simulink model "sampleModel104"  (R2021b)
settings: Solver=VariableStepAuto  StartTime=0.0  StopTime=10.0  RelTol=1e-3
undefined symbols (not defined in the file or in its folder): Newton, Raphson
libraries: simulink x17, slpidlib x1
settings Model: Creator=user  LastModifiedBy=user

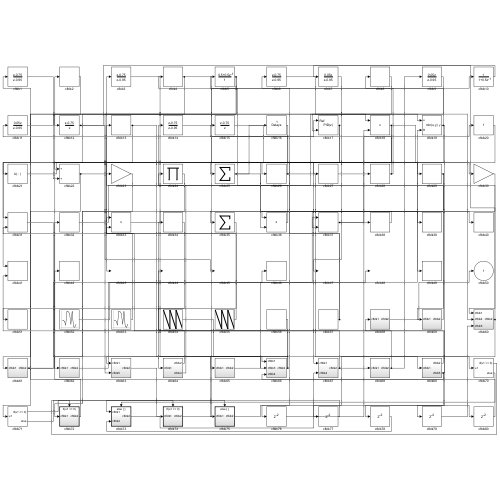
[thumbnail: Simulink's stored preview of the top-level diagram]
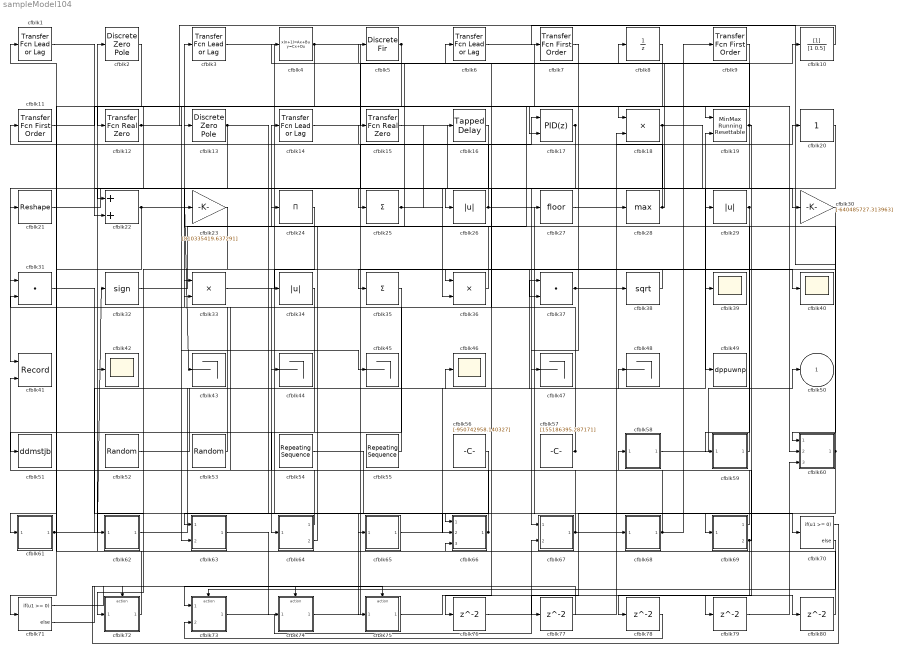
== system sampleModel104 ==
  cfblk{1,3,6,14} (4 alike) : simulink/Discrete/Transfer Fcn Lead or Lag  PoleZ=0.95  ZeroZ=0.75  ICPrevOutput=0.0  ICPrevInput=0.0  DoSatur=off
      settings: SourceProductBaseCode=SL
  cfblk10 : DiscreteFilter  SampleTime=1
  cfblk11 : simulink/Discrete/Transfer Fcn First Order  PoleZ=0.95  ICPrevOutput=0.0  DoSatur=off
  cfblk12 : simulink/Discrete/Transfer Fcn Real Zero  ZeroZ=0.75  ICPrevInput=0.0  DoSatur=off
      settings: SourceProductBaseCode=SL
  cfblk13 : DiscreteZeroPole  Poles=[0 0.5]  Gain=1
  cfblk15 : simulink/Discrete/Transfer Fcn Real Zero  ZeroZ=0.75  ICPrevInput=0.0  DoSatur=off
      settings: SourceProductBaseCode=SL
  cfblk16 : simulink/Discrete/Tapped Delay  vinit=0.0  samptime=-1  NumDelays=1  DelayOrder=Oldest  includeCurrent=off
  cfblk17 : slpidlib/PID Controller (2DOF)  Controller=PID  Form=Parallel  TimeDomain=Discrete-time  UseExternalTs=off  SampleTime=1  IntegratorMethod=Forward Euler  FilterMethod=Forward Euler  ControllerParametersSource=internal  P=1  I=1  D=0  UseFilter=on  N=100  b=1  c=1  TunerSelectOption=Transfer Function Based (PID Tuner App)  InitialConditionSource=internal  InitialConditionForIntegrator=0  InitialConditionForFilter=0  DifferentiatorICPrevScaledInput=0  ExternalReset=none  TrackingMode=off  Kt=1  LimitOutput=off  SatLimitsSource=internal  UpperSaturationLimit=inf  LowerSaturationLimit=-inf  LinearizeAsGain=off  AntiWindupMode=none  Kb=1  POutMin=[]  POutMax=[]  IOutMin=[]  IOutMax=[]  DOutMin=[]  DOutMax=[]  NOutMin=[]  NOutMax=[]  bOutMin=[]  bOutMax=[]  cOutMin=[]  cOutMax=[]  SumOutMin=[]  SumOutMax=[]  SaturationOutMin=[]  SaturationOutMax=[]  PParamMin=[]  PParamMax=[]  IParamMin=[]  IParamMax=[]  DParamMin=[]  DParamMax=[]  NParamMin=[]  NParamMax=[]  bParamMin=[]  bParamMax=[]  cParamMin=[]  cParamMax=[]  KbParamMin=[]  KbParamMax=[]  KtParamMin=[]  KtParamMax=[]  KbOutMin=[]  KbOutMax=[]  KtOutMin=[]  KtOutMax=[]  IntegratorOutMin=[]  IntegratorOutMax=[]  FilterOutMin=[]  FilterOutMax=[]  SumI1OutMin=[]  SumI1OutMax=[]  SumI2OutMin=[]  SumI2OutMax=[]  SumI3OutMin=[]  SumI3OutMax=[]  SumI4OutMin=[]  SumI4OutMax=[]  SumDOutMin=[]  SumDOutMax=[]  Sum1OutMin=[]  Sum1OutMax=[]  Sum2OutMin=[]  Sum2OutMax=[]  Sum3OutMin=[]  Sum3OutMax=[]  DifferentiatorOutMin=[]  DifferentiatorOutMax=[]  FilterDiffOutCoefMin=[]  FilterDiffOutCoefMax=[]  ReciprocalOutMin=[]  ReciprocalOutMax=[]  SumDenOutMin=[]  SumDenOutMax=[]  SumNumOutMin=[]  SumNumOutMax=[]  DivideOutMin=[]  DivideOutMax=[]  UdiffTsProdOutMin=[]  UdiffTsProdOutMax=[]  NTsProdOutMin=[]  NTsProdOutMax=[]  UintegralTsProdOutMin=[]  UintegralTsProdOutMax=[]  UngainTsProdOutMin=[]  UngainTsProdOutMax=[]  IntegratorContinuousStateAttributes=''  IntegratorStateMustResolveToSignalObject=off  IntegratorRTWStateStorageClass=Auto  FilterContinuousStateAttributes=''  FilterStateMustResolveToSignalObject=off  FilterRTWStateStorageClass=Auto  ParallelPVariant=InternalParameters  IdealPVariant=Disabled  IVariant=InternalParameters  DVariant=InternalParameters  bVariant=InternalParameters  cVariant=InternalParameters  IntegratorVariant=Discrete  SatVariant=Disabled  AWVariant=Passthrough  PCopyVariant=Disabled  TRVariant=Disabled  FdbkBlocksVariant=Forward  IdealPFdbkVariant=Disabled  SatFdbkVariant=Disabled  DerivativeFilterVariant=ForwardEulerFilter  NVariant=InternalParameters  NCopyVariant=Disabled  FilterICVariant=InternalICsFilter  IntegratorICVariant=InternalICs  ExternalResetVariant=Disabled  TRSumVariant=Passthrough  SumFdbkVariant=Disabled  SumVariant=Sum_PID  TsampFilterVariant=InternalTs  TsampNgainVariant=Passthrough  TsampIntegralVariant=Passthrough  ExternalSaturationOutDataTypeStr=Inherit: Same as second input
      settings: SourceProductBaseCode=SL
  cfblk18 : Product  Inputs=**
  cfblk19 : simulink/Math Operations/MinMax Running Resettable  Function=min  vinit=0.0
  cfblk2 : DiscreteZeroPole  Poles=[0 0.5]  Gain=1
  cfblk20 : simulink/Math Operations/Slider Gain  gain=1  low=0  high=2
  cfblk21 : Reshape
  cfblk22 : Sum
  cfblk23 : Gain  Gain=[810335419.637291]
  cfblk24 : Product  Inputs=*
  cfblk25 : Sum  Inputs=+
  cfblk26 : Abs
  cfblk27 : Rounding
  cfblk28 : MinMax  Function=max
  cfblk29 : Abs
  cfblk30 : Gain  Gain=[-640485727.313963]
  cfblk31 : DotProduct  InputSameDT=on  OutDataTypeStr=Inherit: Inherit via internal rule
  cfblk32 : Signum
  cfblk33 : Product
  cfblk34 : Abs
  cfblk35 : Sum  Inputs=+
  cfblk36 : Product  Inputs=**
  cfblk37 : DotProduct  InputSameDT=on  OutDataTypeStr=Inherit: Inherit via internal rule
  cfblk38 : Sqrt  SaturateOnIntegerOverflow=on
  cfblk{39..40,42,46} (4 alike) : Scope
  cfblk4 : DiscreteStateSpace
  cfblk41 : Record  FileSettingsInternal="{\"entries\":[{\"content\":{\"excelSettings\":{\"content\":{},\"type\":\"Streamout.ExcelSettings\"}},\"type\":\"Streamout.FileSettingStorage\",\"uuid\":\"84cf82fa-35bb-4254-a1fc-1f6b5955f86e\"}],\"packageUris\":[\"http://schema.mathworks.com/mf0/streamout_blocks/R2020a\"],\"version\":\"1.0\"}"  Layout=[1 1]  SignalsInternal="{\"entries\":[{\"content\":{\"signals\":[{\"content\":{\"blockPath\":[\"sampleModel104/cfblk41\"],\"channel\":[],\"dimensions\":[1],\"domain\":\"sampleModel104/cfblk41\",\"lineColor\":\"#a2142f\",\"plots\":[1],\"port\":1,\"sid\":[\"\"],\"signalID\":3732,\"signalName\":\"cfblk16\"},\"type\":\"RecordBlkView.Signal\",\"uuid\":\"75152f1e-4c02-4af2-84cf-784db9ba61d4\"},{\"content\":{\"blockPath\":[\"sampleModel104/cfblk41\"],\"channel\":[],\"dimensions\":[1],\"domain\":\"sampleModel104/cfblk41\",\"lineColor\":\"#139fff\",\"plots\":[1],\"port\":2,\"sid\":[\"\"],\"signalID\":3736,\"signalName\":\"cfblk66\"},\"type\":\"RecordBlkView.Signal\",\"uuid\":\"7964c5ee-3da1-484c-b3b6-d9e0f74eaa61\"}]},\"type\":\"RecordBlkView.InputSignals\",\"uuid\":\"6aa1200e-81fa-4e57-8f02-0c25f67a03be\"}],\"packageUris\":[\"http://schema.mathworks.com/mf0/streamout_blocks/R2020a\"],\"version\":\"1.0\"}"  VisualizationBindings="{\"xyplotplugin\":{\"info\":[{\"series\":[{\"bindingParametersList\":[{\"parameter\":\"X-Axis\",\"signalID\":3732,\"signalName\":\"cfblk16\"},{\"parameter\":\"Y-Axis\",\"signalID\":3736,\"signalName\":\"cfblk66\"}],\"seriesID\":3868}],\"subplotID\":1}]}}"  CompatibilityTag=XY
  cfblk{43..45,47..48} (5 alike) : Terminator
  cfblk49 : ToWorkspace  VariableName=dppuwnp  SaveFormat=Timeseries  SampleTime=-1
  cfblk5 : DiscreteFir  SampleTime=1
  cfblk51 : ToWorkspace  VariableName=ddmstjb  SaveFormat=Timeseries  SampleTime=-1
  cfblk52 : RandomNumber  Mean=[-16667.436370]  Variance=[47383.574054]  Seed=[56841479.000000]  SampleTime=0.1
  cfblk53 : RandomNumber  Mean=[25600.008098]  Variance=[37838.678242]  Seed=[330531999.000000]  SampleTime=0.1
  cfblk54 : simulink/Sources/Repeating Sequence  rep_seq_t=[0 2]  rep_seq_y=[249633370.551990, -336076107.817194]
  cfblk55 : simulink/Sources/Repeating Sequence  rep_seq_t=[0 2]  rep_seq_y=[799947842.512021, 579171463.259229]
  cfblk56 : Constant  Value=[-950742958.140327]  SampleTime=1
  cfblk57 : Constant  Value=[155186395.287171]  SampleTime=1
  cfblk58 : Subsystem
  cfblk59 : Subsystem
  cfblk60 : Subsystem
  cfblk61 : Subsystem
  cfblk62 : Subsystem
  cfblk63 : Subsystem
  cfblk64 : Subsystem
  cfblk65 : Subsystem
  cfblk66 : Subsystem
  cfblk67 : Subsystem
  cfblk68 : Subsystem
  cfblk69 : Subsystem
  cfblk7 : simulink/Discrete/Transfer Fcn First Order  PoleZ=0.95  ICPrevOutput=0.0  DoSatur=off
  cfblk70 : If  IfExpression=u1 >= 0  SampleTime=1
  cfblk71 : If  IfExpression=u1 >= 0  SampleTime=1
  cfblk72 : Subsystem  TreatAsAtomicUnit=on
  cfblk73 : Subsystem  TreatAsAtomicUnit=on
  cfblk74 : Subsystem  TreatAsAtomicUnit=on
  cfblk75 : Subsystem  TreatAsAtomicUnit=on
  cfblk{76..80} (5 alike) : Delay  SampleTime=1
  cfblk8 : UnitDelay  HasFrameUpgradeWarning=on
  cfblk9 : simulink/Discrete/Transfer Fcn First Order  PoleZ=0.95  ICPrevOutput=0.0  DoSatur=off
  cfblk50 : Outport
  wires:
  cfblk18/1 -> cfblk67/1(cfblk1), cfblk30/1, cfblk23/1
  cfblk16/1 -> cfblk41/1
  cfblk33/1 -> cfblk40/1
  cfblk32/1 -> cfblk19/1
  cfblk73/1(cfblk2) -> cfblk67/2(cfblk4)
  cfblk3/1 -> cfblk66/1(cfblk1)
  cfblk74/1(cfblk2) -> cfblk17/1
  cfblk17/1 -> cfblk31/1, cfblk76/1
  cfblk66/1(cfblk2) -> cfblk41/2, cfblk63/1(cfblk1)
  cfblk27/1 -> cfblk28/1
  cfblk72/1(cfblk2) -> cfblk2/1
  cfblk26/1 -> cfblk69/1(cfblk1), cfblk15/1
  cfblk36/1 -> cfblk3/1
  cfblk55/1 -> cfblk31/2
  cfblk7/1 -> cfblk47/1
  cfblk1/1 -> cfblk27/1
  cfblk59/1(cfblk2) -> cfblk14/1
  cfblk28/1 -> cfblk11/1, cfblk8/1
  cfblk19/1 -> cfblk26/1, cfblk4/1, cfblk79/1
  cfblk69/1(cfblk2) -> cfblk34/1
  cfblk69/2(cfblk5) -> cfblk58/1(cfblk1), cfblk66/3(cfblk4), cfblk78/1
  cfblk2/1 -> cfblk12/1
  cfblk12/1 -> cfblk60/1(cfblk1), cfblk45/1
  cfblk20/1 -> cfblk25/1
  cfblk61/1(cfblk2) -> cfblk32/1, cfblk46/1
  cfblk9/1 -> cfblk17/2
  cfblk54/1 -> cfblk66/2(cfblk3)
  cfblk52/1 -> cfblk19/2
  cfblk57/1 -> cfblk6/1, cfblk24/1
  cfblk56/1 -> cfblk75/1(cfblk1)
  cfblk60/1(cfblk2) -> cfblk5/1, cfblk77/1
  cfblk4/1 -> cfblk21/1, cfblk36/2
  cfblk68/1(cfblk2) -> cfblk44/1, cfblk9/1
  cfblk15/1 -> cfblk49/1
  cfblk65/1(cfblk2) -> cfblk48/1
  cfblk22/1 -> cfblk43/1, cfblk71/1
  cfblk38/1 -> cfblk35/1
  cfblk11/1 -> cfblk18/1
  cfblk53/1 -> cfblk13/1
  cfblk6/1 -> cfblk60/2(cfblk4)
  cfblk5/1 -> cfblk61/1(cfblk1), cfblk63/2(cfblk5)
  cfblk31/1 -> cfblk65/1(cfblk1)
  cfblk13/1 -> cfblk70/1, cfblk22/2
  cfblk25/1 -> cfblk39/1, cfblk16/1
  cfblk21/1 -> cfblk29/1
  cfblk62/1(cfblk2) -> cfblk37/1
  cfblk64/1(cfblk2) -> cfblk33/1
  cfblk30/1 -> cfblk36/1
  cfblk29/1 -> cfblk37/2, cfblk59/1(cfblk1)
  cfblk34/1 -> cfblk51/1
  cfblk37/1 -> cfblk38/1, cfblk20/1
  cfblk24/1 -> cfblk62/1(cfblk1)
  cfblk35/1 -> cfblk64/1(cfblk1)
  cfblk63/1(cfblk2) -> cfblk74/1(cfblk1)
  cfblk64/2(cfblk4) -> cfblk33/2
  cfblk8/1 -> cfblk22/1
  cfblk67/1(cfblk2) -> cfblk68/1(cfblk1), cfblk42/1
  cfblk23/1 -> cfblk72/1(cfblk1)
  cfblk14/1 -> cfblk10/1
  cfblk10/1 -> cfblk7/1
  cfblk58/1(cfblk2) -> cfblk50/1
  cfblk70/1 -> cfblk72/Action
  cfblk70/2 -> cfblk73/Action
  cfblk71/1 -> cfblk74/Action
  cfblk71/2 -> cfblk75/Action
  cfblk76/1 -> cfblk18/2
  cfblk77/1 -> cfblk73/1(cfblk1)
  cfblk78/1 -> cfblk73/2(cfblk4)
  cfblk79/1 -> cfblk60/3(cfblk5)
  cfblk75/1(cfblk2) -> cfblk80/1
  cfblk80/1 -> cfblk1/1

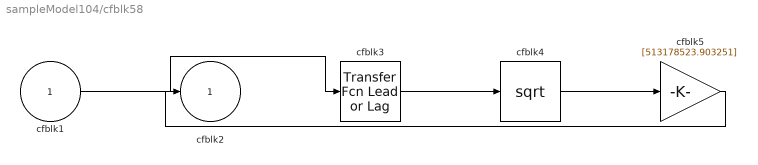
== system sampleModel104/cfblk58 ==
  cfblk1 : Inport
  cfblk3 : simulink/Discrete/Transfer Fcn Lead or Lag  PoleZ=0.95  ZeroZ=0.75  ICPrevOutput=0.0  ICPrevInput=0.0  DoSatur=off
      settings: SourceProductBaseCode=SL
  cfblk4 : Sqrt  SaturateOnIntegerOverflow=on
  cfblk5 : Gain  Gain=[513178523.903251]
  cfblk2 : Outport
  wires:
  cfblk3/1 -> cfblk4/1
  cfblk4/1 -> cfblk5/1
  cfblk1/1 -> cfblk3/1
  cfblk5/1 -> cfblk2/1

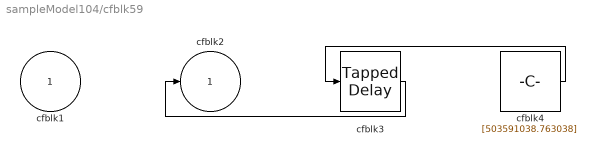
== system sampleModel104/cfblk59 ==
  cfblk1 : Inport
  cfblk3 : simulink/Discrete/Tapped Delay  vinit=0.0  samptime=-1  NumDelays=1  DelayOrder=Oldest  includeCurrent=off
  cfblk4 : Constant  Value=[503591038.763038]  SampleTime=1
  cfblk2 : Outport
  wires:
  cfblk4/1 -> cfblk3/1
  cfblk3/1 -> cfblk2/1

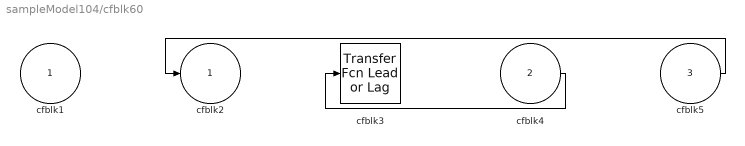
== system sampleModel104/cfblk60 ==
  cfblk1 : Inport
  cfblk4 : Inport  Port=2
  cfblk5 : Inport  Port=3
  cfblk3 : simulink/Discrete/Transfer Fcn Lead or Lag  PoleZ=0.95  ZeroZ=0.75  ICPrevOutput=0.0  ICPrevInput=0.0  DoSatur=off
      settings: SourceProductBaseCode=SL
  cfblk2 : Outport
  wires:
  cfblk5/1 -> cfblk2/1
  cfblk4/1 -> cfblk3/1

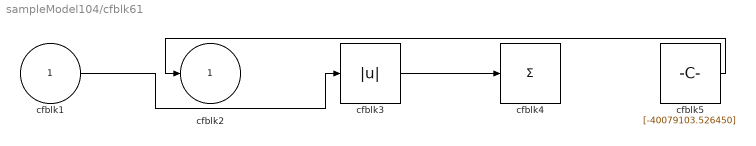
== system sampleModel104/cfblk61 ==
  cfblk1 : Inport
  cfblk3 : Abs
  cfblk4 : Sum  Inputs=+
  cfblk5 : Constant  Value=[-40079103.526450]  SampleTime=1
  cfblk2 : Outport
  wires:
  cfblk5/1 -> cfblk2/1
  cfblk1/1 -> cfblk3/1
  cfblk3/1 -> cfblk4/1

== system sampleModel104/cfblk62 ==
  cfblk1 : Inport
  cfblk3 : UnitDelay  HasFrameUpgradeWarning=on
  cfblk4 : Trigonometry
  cfblk2 : Outport
  wires:
  cfblk4/1 -> cfblk2/1
  cfblk1/1 -> cfblk3/1
  cfblk3/1 -> cfblk4/1

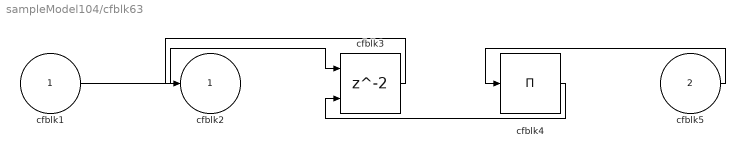
== system sampleModel104/cfblk63 ==
  cfblk1 : Inport
  cfblk5 : Inport  Port=2
  cfblk3 : Delay  ShowEnablePort=on  SampleTime=1
      settings: InputPortMap=u0,e6
  cfblk4 : Product  Inputs=*
  cfblk2 : Outport
  wires:
  cfblk1/1 -> cfblk3/1
  cfblk4/1 -> cfblk3/2
  cfblk5/1 -> cfblk4/1
  cfblk3/1 -> cfblk2/1

== system sampleModel104/cfblk64 ==
  cfblk1 : Inport
  cfblk3 : Signum
  cfblk2 : Outport
  cfblk4 : Outport  Port=2
  wires:
  cfblk1/1 -> cfblk2/1, cfblk3/1
  cfblk3/1 -> cfblk4/1

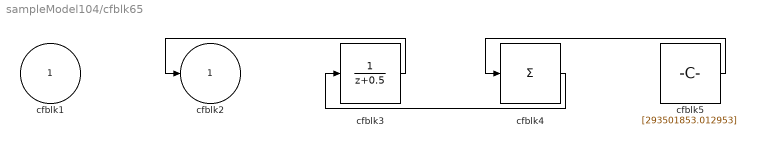
== system sampleModel104/cfblk65 ==
  cfblk1 : Inport
  cfblk3 : DiscreteTransferFcn  SampleTime=1
  cfblk4 : Sum  Inputs=+
  cfblk5 : Constant  Value=[293501853.012953]  SampleTime=1
  cfblk2 : Outport
  wires:
  cfblk3/1 -> cfblk2/1
  cfblk5/1 -> cfblk4/1
  cfblk4/1 -> cfblk3/1

== system sampleModel104/cfblk66 ==
  cfblk1 : Inport
  cfblk3 : Inport  Port=2
  cfblk4 : Inport  Port=3
  cfblk2 : Outport
  wires:
  cfblk1/1 -> cfblk2/1

== system sampleModel104/cfblk67 ==
  cfblk1 : Inport
  cfblk4 : Inport  Port=2
  cfblk3 : Product
  cfblk2 : Outport
  wires:
  cfblk1/1 -> cfblk2/1
  cfblk4/1 -> cfblk3/1, cfblk3/2

== system sampleModel104/cfblk68 ==
  cfblk1 : Inport
  cfblk3 : Product  Inputs=**
  cfblk2 : Outport
  wires:
  cfblk3/1 -> cfblk2/1
  cfblk1/1 -> cfblk3/1, cfblk3/2

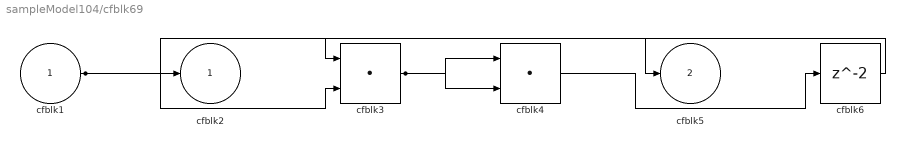
== system sampleModel104/cfblk69 ==
  cfblk1 : Inport
  cfblk3 : DotProduct  InputSameDT=on  OutDataTypeStr=Inherit: Inherit via internal rule
  cfblk4 : DotProduct  InputSameDT=on  OutDataTypeStr=Inherit: Inherit via internal rule
  cfblk6 : Delay  SampleTime=1
  cfblk2 : Outport
  cfblk5 : Outport  Port=2
  wires:
  cfblk1/1 -> cfblk2/1, cfblk3/2, cfblk5/1
  cfblk3/1 -> cfblk4/1, cfblk4/2
  cfblk4/1 -> cfblk6/1
  cfblk6/1 -> cfblk3/1

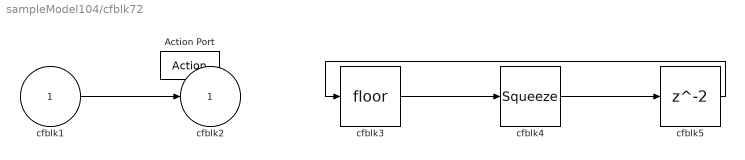
== system sampleModel104/cfblk72 ==
  cfblk1 : Inport
  Action Port : ActionPort  ActionPortLabel=if(u1 >= 0)
  cfblk3 : Rounding
  cfblk4 : Squeeze
  cfblk5 : Delay
  cfblk2 : Outport
  wires:
  cfblk1/1 -> cfblk2/1
  cfblk3/1 -> cfblk4/1
  cfblk4/1 -> cfblk5/1
  cfblk5/1 -> cfblk3/1

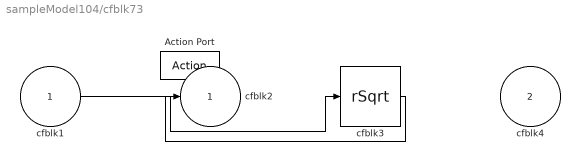
== system sampleModel104/cfblk73 ==
  cfblk1 : Inport
  cfblk4 : Inport  Port=2
  Action Port : ActionPort  ActionPortLabel=else
  cfblk3 : Sqrt  Operator=rSqrt  AlgorithmType=Newton-Raphson  SaturateOnIntegerOverflow=on
  cfblk2 : Outport
  wires:
  cfblk1/1 -> cfblk3/1
  cfblk3/1 -> cfblk2/1

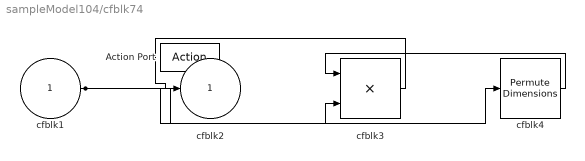
== system sampleModel104/cfblk74 ==
  cfblk1 : Inport
  Action Port : ActionPort  ActionPortLabel=if(u1 >= 0)
  cfblk3 : Product
  cfblk4 : PermuteDimensions
  cfblk2 : Outport
  wires:
  cfblk1/1 -> cfblk4/1, cfblk3/2
  cfblk3/1 -> cfblk2/1
  cfblk4/1 -> cfblk3/1

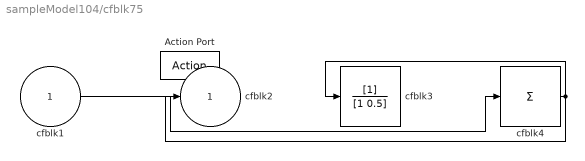
== system sampleModel104/cfblk75 ==
  cfblk1 : Inport
  Action Port : ActionPort  ActionPortLabel=else
  cfblk3 : DiscreteFilter
  cfblk4 : Sum  Inputs=+
  cfblk2 : Outport
  wires:
  cfblk1/1 -> cfblk4/1
  cfblk4/1 -> cfblk2/1, cfblk3/1
